simulink model "P4_Wk3"  (R2024b)
settings: Solver=ode4  StartTime=0.0  StopTime=3000  FixedStep=1  RelTol=1e-3
undefined symbols (not defined in the file or in its folder): CD, datBat, datMotor, TD, track
libraries: slpidlib x1
settings Model: Creator=brekw  LastModifiedBy=brekw
settings DebuggingCC: AlgebraicLoopMsg=none

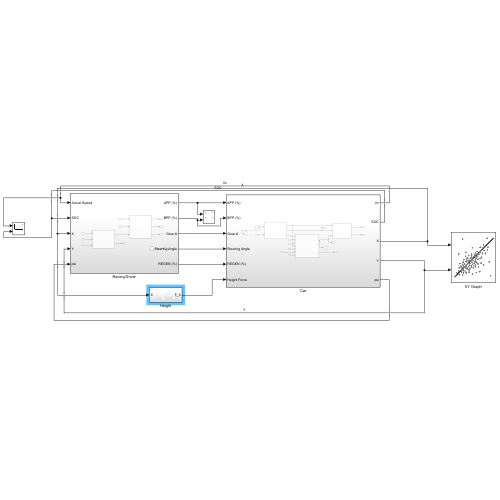
[thumbnail: Simulink's stored preview of the top-level diagram]
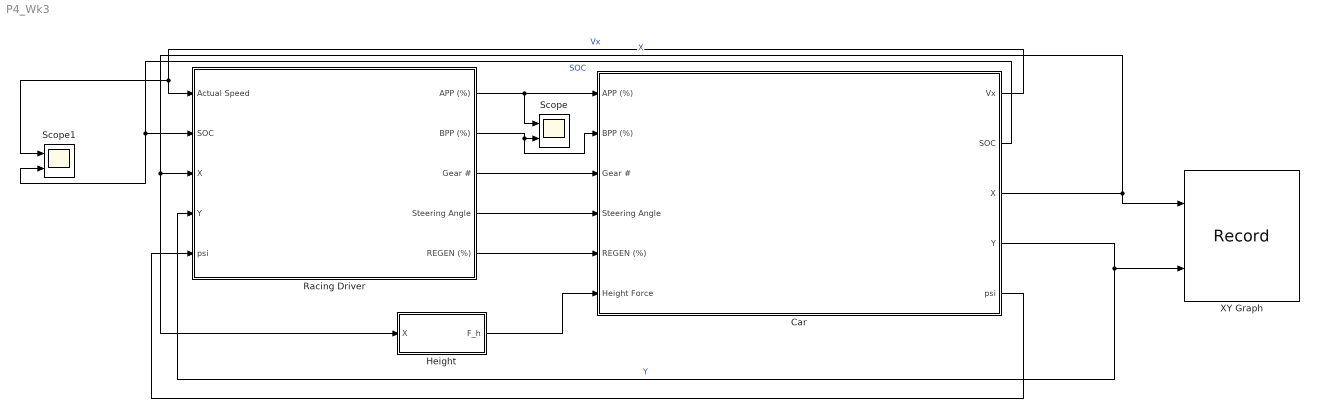
== system P4_Wk3 ==
  Car : Subsystem
  Height : Subsystem
  Racing Driver : Subsystem
  Scope : Scope  NumInputPorts=2
  Scope1 : Scope  NumInputPorts=2
  XY Graph : Record  FileSettingsInternal="{\"entries\":[{\"content\":{\"excelSettings\":{\"content\":{},\"type\":\"Streamout.ExcelSettings\"}},\"type\":\"Streamout.FileSettingStorage\",\"uuid\":\"\"}],\"packageUris\":[\"http:\\/\\/schema.mathworks.com\\/mf0\\/streamout_blocks\\/R2020a\"],\"version\":\"1.0\"}"  Layout=[1 1]  SignalsInternal="{\"entries\":[{\"content\":{\"signals\":[{\"content\":{\"blockPath\":[],\"dimensions\":[1],\"domain\":\"\",\"lineColor\":\"#a2142f\",\"plots\":[ 1 ],\"port\":1,\"sid\":[\"\"],\"signalID\":1,\"signalName\":\"X\"},\"type\":\"RecordBlkView.Signal\",\"uuid\":\"\"},{\"content\":{\"blockPath\":[],\"dimensions\":[1],\"domain\":\"\",\"lineColor\":\"#139fff\",\"plots\":[ 1 ],\"port\":2,\"sid\":[\"\"],\"signalID\":2,\"signalName\":\"Y\"},\"type\":\"RecordBlkView.Signal\",\"uuid\":\"\"}]},\"type\":\"RecordBlkView.InputSignals\",\"uuid\":\"\"}],\"packageUris\":[\"http:\\/\\/schema.mathworks.com\\/mf0\\/streamout_blocks\\/R2020a\"],\"version\":\"1.0\"}"  VisualizationBindings="{\"xyplotplugin\":{\"info\":[{\"series\":[{\"bindingParametersList\":[{\"parameter\":\"X-Axis\",\"signalID\":1,\"signalName\":\"X\"},{\"parameter\":\"Y-Axis\",\"signalID\":2,\"signalName\":\"Y\"}],\"seriesID\":0}],\"subplotID\":1}]}}"  CompatibilityTag=XY
  wires:
  Car/3(X) -> XY Graph/1, Height/1(X), Racing Driver/3(X)  "X"
  Car/4(Y) -> XY Graph/2, Racing Driver/4(Y)  "Y"
  Racing Driver/4(Steering Angle) -> Car/4(Steering Angle)
  Racing Driver/3(Gear #) -> Car/3(Gear #)
  Racing Driver/2(BPP (%)) -> Car/2(BPP (%)), Scope/2
  Racing Driver/1(APP (%)) -> Scope/1, Car/1(APP (%))
  Car/1(Vx) -> Scope1/1, Racing Driver/1(Actual Speed)  "Vx"
  Car/2(SOC) -> Scope1/2, Racing Driver/2(SOC)  "SOC"
  Racing Driver/5(REGEN (%)) -> Car/5(REGEN (%))
  Car/5(psi) -> Racing Driver/5(psi)
  Height/1(F_h) -> Car/6(Height Force)

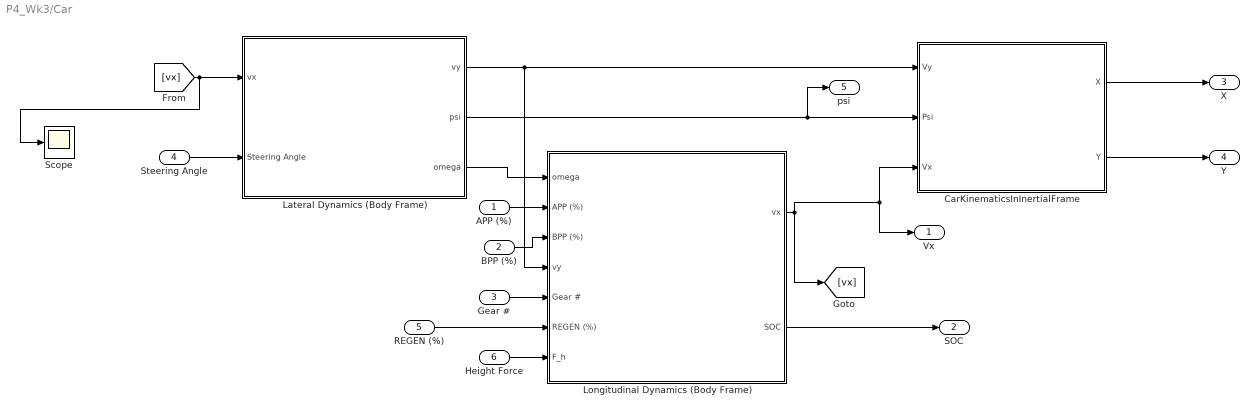
== system P4_Wk3/Car ==
  APP (%) : Inport
  BPP (%) : Inport  Port=2
  Gear # : Inport  Port=3
  Steering Angle : Inport  Port=4
  REGEN (%) : Inport  Port=5
  Height Force : Inport  Port=6
  CarKinematicsInInertialFrame : Subsystem
  Lateral Dynamics (Body Frame) : Subsystem
  Longitudinal Dynamics (Body Frame) : Subsystem
  Scope : Scope
  Vx : Outport
  SOC : Outport  Port=2
  X : Outport  Port=3
  Y : Outport  Port=4
  psi : Outport  Port=5
  wires:
  CarKinematicsInInertialFrame/1(X) -> X/1
  CarKinematicsInInertialFrame/2(Y) -> Y/1
  Lateral Dynamics (Body Frame)/1(vy) -> CarKinematicsInInertialFrame/1(Vy), Longitudinal Dynamics (Body Frame)/4(vy)
  Lateral Dynamics (Body Frame)/2(psi) -> psi/1, CarKinematicsInInertialFrame/2(Psi)
  Steering Angle/1 -> Lateral Dynamics (Body Frame)/2(Steering Angle)
  Longitudinal Dynamics (Body Frame)/1(vx) -> CarKinematicsInInertialFrame/3(Vx), Vx/1, [vx]
  Longitudinal Dynamics (Body Frame)/2(SOC) -> SOC/1
  Lateral Dynamics (Body Frame)/3(omega) -> Longitudinal Dynamics (Body Frame)/1(omega)
  [vx] -> Scope/1, Lateral Dynamics (Body Frame)/1(vx)
  Gear #/1 -> Longitudinal Dynamics (Body Frame)/5(Gear #)
  BPP (%)/1 -> Longitudinal Dynamics (Body Frame)/3(BPP (%))
  APP (%)/1 -> Longitudinal Dynamics (Body Frame)/2(APP (%))
  REGEN (%)/1 -> Longitudinal Dynamics (Body Frame)/6(REGEN (%))
  Height Force/1 -> Longitudinal Dynamics (Body Frame)/7(F_h)

== system P4_Wk3/Height ==
  X : Inport
  Constant : Constant  Value=CD.Mass
  Elevation Profile : MATLAB Function  TreatAsAtomicUnit=on
  Height Force : MATLAB Function  TreatAsAtomicUnit=on
  Scope : Scope
  F_h : Outport
  wires:
  Height Force/1(F) -> F_h/1
  X/1 -> Elevation Profile/1(x)
  Elevation Profile/2(theta) -> Height Force/2(theta)
  Constant/1 -> Height Force/1(m)
  Elevation Profile/1(h) -> Scope/1

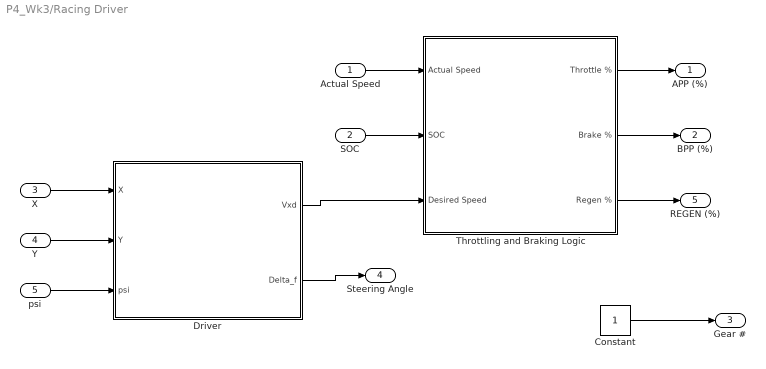
== system P4_Wk3/Racing Driver ==
  Actual Speed : Inport
  SOC : Inport  Port=2
  X : Inport  Port=3
  Y : Inport  Port=4
  psi : Inport  Port=5
  Constant : Constant
  Driver : Subsystem
  Throttling and Braking Logic : Subsystem
  APP (%) : Outport
  BPP (%) : Outport  Port=2
  Gear # : Outport  Port=3
  Steering Angle : Outport  Port=4
  REGEN (%) : Outport  Port=5
  wires:
  Constant/1 -> Gear #/1
  Driver/2(Delta_f) -> Steering Angle/1
  Driver/1(Vxd) -> Throttling and Braking Logic/3(Desired Speed)
  Actual Speed/1 -> Throttling and Braking Logic/1(Actual Speed)
  SOC/1 -> Throttling and Braking Logic/2(SOC)
  Throttling and Braking Logic/1(Throttle %) -> APP (%)/1
  Throttling and Braking Logic/2(Brake %) -> BPP (%)/1
  X/1 -> Driver/1(X)
  Y/1 -> Driver/2(Y)
  Throttling and Braking Logic/3(Regen %) -> REGEN (%)/1
  psi/1 -> Driver/3(psi)

== system P4_Wk3/Car/CarKinematicsInInertialFrame ==
  Vy : Inport
  Psi : Inport  Port=2
  Vx : Inport  Port=3
  Integrator : Integrator  InitialCondition=CD.X0
  Integrator1 : Integrator  InitialCondition=CD.Y0
  Transformation Matrix : MATLAB Function  TreatAsAtomicUnit=on
  Xdot Out : ToWorkspace  VariableName=X  SaveFormat=Timeseries  SampleTime=-1
  Ydot Out : ToWorkspace  VariableName=Y  SaveFormat=Timeseries  SampleTime=-1
  X : Outport
  Y : Outport  Port=2
  wires:
  Transformation Matrix/2(Ydot) -> Integrator1/1
  Vy/1 -> Transformation Matrix/2(vy)
  Integrator/1 -> Xdot Out/1, X/1
  Psi/1 -> Transformation Matrix/3(psi)
  Integrator1/1 -> Ydot Out/1, Y/1
  Transformation Matrix/1(Xdot) -> Integrator/1
  Vx/1 -> Transformation Matrix/1(vx)

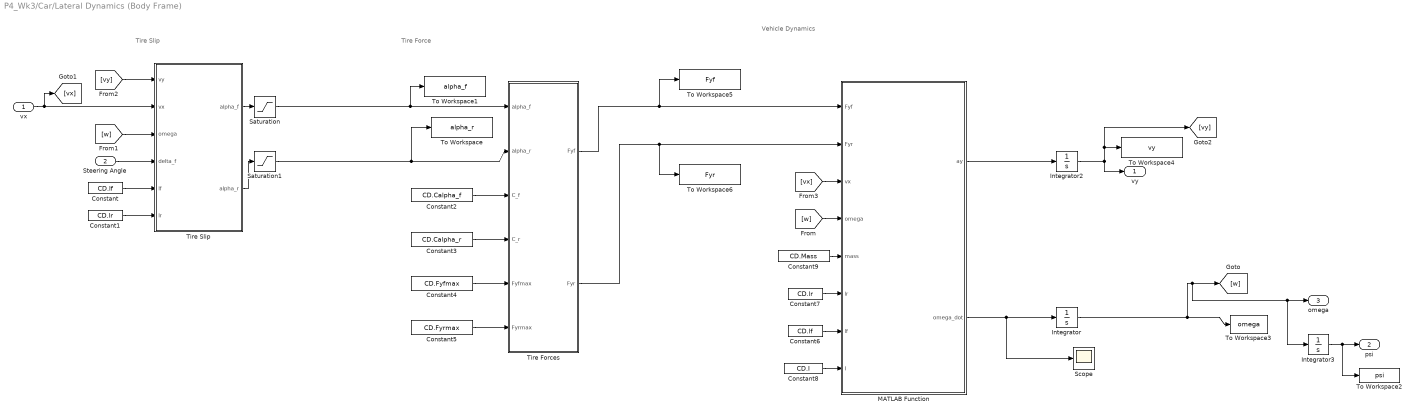
== system P4_Wk3/Car/Lateral Dynamics (Body Frame) ==
  note: Tire Slip
  note: Vehicle Dynamics
  note: Tire Force
  vx : Inport
  Steering Angle : Inport  Port=2
  Constant : Constant  Value=CD.lf
  Constant1 : Constant  Value=CD.lr
  Constant2 : Constant  Value=CD.Calpha_f
  Constant3 : Constant  Value=CD.Calpha_r
  Constant4 : Constant  Value=CD.Fyfmax
  Constant5 : Constant  Value=CD.Fyrmax
  Constant6 : Constant  Value=CD.lf
  Constant7 : Constant  Value=CD.lr
  Constant8 : Constant  Value=CD.I
  Constant9 : Constant  Value=CD.Mass
  Integrator : Integrator  InitialCondition=CD.omega0
  Integrator2 : Integrator  InitialCondition=CD.vy0
  Integrator3 : Integrator  InitialCondition=CD.psi0
  MATLAB Function : MATLAB Function  TreatAsAtomicUnit=on
  Saturation : Saturate  UpperLimit=0.01579  LowerLimit=-0.01579
  Saturation1 : Saturate  UpperLimit=0.01579  LowerLimit=-0.01579
  Scope : Scope
  Tire Forces : MATLAB Function  TreatAsAtomicUnit=on
  Tire Slip : MATLAB Function  TreatAsAtomicUnit=on
  To Workspace : ToWorkspace  VariableName=alpha_r  SaveFormat=Timeseries  SampleTime=-1
  To Workspace1 : ToWorkspace  VariableName=alpha_f  SaveFormat=Timeseries  SampleTime=-1
  To Workspace2 : ToWorkspace  VariableName=psi  SaveFormat=Timeseries  SampleTime=-1
  To Workspace3 : ToWorkspace  VariableName=omega  SaveFormat=Timeseries  SampleTime=-1
  To Workspace4 : ToWorkspace  VariableName=vy  SaveFormat=Timeseries  SampleTime=-1
  To Workspace5 : ToWorkspace  VariableName=Fyf  SaveFormat=Timeseries  SampleTime=-1
  To Workspace6 : ToWorkspace  VariableName=Fyr  SaveFormat=Timeseries  SampleTime=-1
  vy : Outport
  psi : Outport  Port=2
  omega : Outport  Port=3
  wires:
  MATLAB Function/2(omega_dot) -> Scope/1, Integrator/1
  Integrator/1 -> omega/1, Integrator3/1, [w], To Workspace3/1
  Integrator2/1 -> To Workspace4/1, [vy], vy/1
  Integrator3/1 -> psi/1, To Workspace2/1
  [w] -> MATLAB Function/4(omega)
  MATLAB Function/1(ay) -> Integrator2/1
  [vy] -> Tire Slip/1(vy)
  Saturation/1 -> To Workspace1/1, Tire Forces/1(alpha_f)
  Saturation1/1 -> To Workspace/1, Tire Forces/2(alpha_r)
  [w] -> Tire Slip/3(omega)
  Steering Angle/1 -> Tire Slip/4(delta_f)
  Tire Slip/1(alpha_f) -> Saturation/1
  Tire Slip/2(alpha_r) -> Saturation1/1
  vx/1 -> [vx], Tire Slip/2(vx)
  [vx] -> MATLAB Function/3(vx)
  Tire Forces/1(Fyf) -> To Workspace5/1, MATLAB Function/1(Fyf)
  Tire Forces/2(Fyr) -> To Workspace6/1, MATLAB Function/2(Fyr)
  Constant/1 -> Tire Slip/5(lf)
  Constant1/1 -> Tire Slip/6(lr)
  Constant2/1 -> Tire Forces/3(C_f)
  Constant3/1 -> Tire Forces/4(C_r)
  Constant4/1 -> Tire Forces/5(Fyfmax)
  Constant5/1 -> Tire Forces/6(Fyrmax)
  Constant7/1 -> MATLAB Function/6(lr)
  Constant6/1 -> MATLAB Function/7(lf)
  Constant8/1 -> MATLAB Function/8(I)
  Constant9/1 -> MATLAB Function/5(mass)

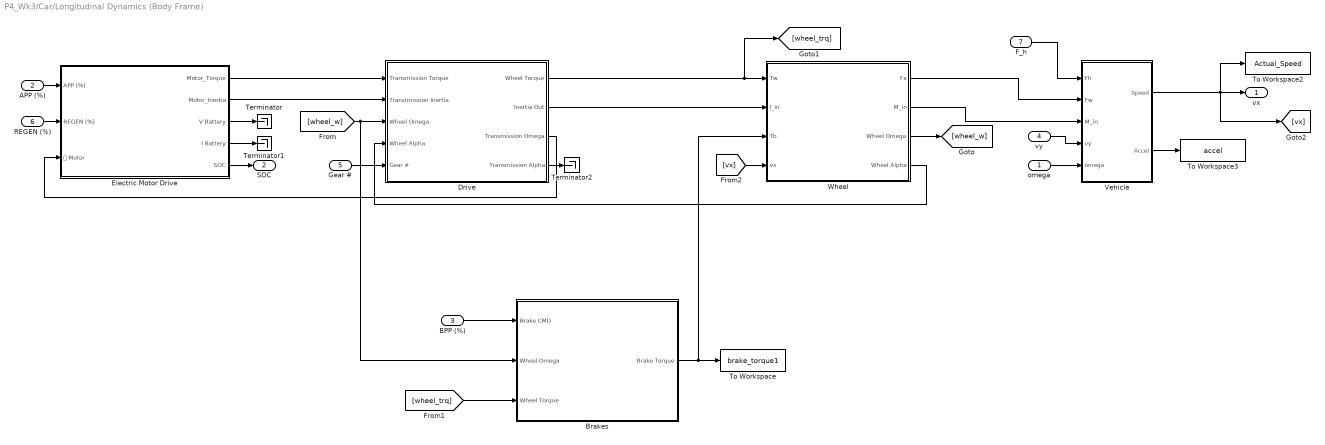
== system P4_Wk3/Car/Longitudinal Dynamics (Body Frame) ==
  omega : Inport
  APP (%) : Inport  Port=2
  BPP (%) : Inport  Port=3
  vy : Inport  Port=4
  Gear # : Inport  Port=5
  REGEN (%) : Inport  Port=6
  F_h : Inport  Port=7
  Brakes : Subsystem
  Drive : Subsystem
  Electric Motor Drive : Subsystem
  Terminator : Terminator
  Terminator1 : Terminator
  Terminator2 : Terminator
  To Workspace : ToWorkspace  VariableName=brake_torque1  SaveFormat=Timeseries  SampleTime=-1
  To Workspace2 : ToWorkspace  VariableName=Actual_Speed  SaveFormat=Timeseries  SampleTime=-1
  To Workspace3 : ToWorkspace  VariableName=accel  SaveFormat=Timeseries  SampleTime=-1
  Vehicle : Subsystem
  Wheel : Subsystem
  vx : Outport
  SOC : Outport  Port=2
  wires:
  Drive/4(Transmission Alpha) -> Terminator2/1
  Drive/2(Inertia Out) -> Wheel/2(I_in)
  [wheel_trq] -> Brakes/3(Wheel Torque)
  Electric Motor Drive/3(V Battery) -> Terminator/1
  Electric Motor Drive/2(Motor_Inertia) -> Drive/2(Transimission Inertia)
  Electric Motor Drive/1(Motor_Torque) -> Drive/1(Transmission Torque)
  Electric Motor Drive/5(SOC) -> SOC/1
  Electric Motor Drive/4(I Battery) -> Terminator1/1
  Wheel/3(Wheel Omega) -> [wheel_w]
  Drive/1(Wheel Torque) -> [wheel_trq], Wheel/1(Tw)
  [wheel_w] -> Brakes/2(Wheel Omega), Drive/3(Wheel Omega)
  BPP (%)/1 -> Brakes/1(Brake CMD)
  Drive/3(Transmission Omega) -> Electric Motor Drive/3(𝜔 Motor)
  Brakes/1(Brake Torque) -> To Workspace/1, Wheel/3(Tb)
  Wheel/2(M_in) -> Vehicle/3(M_in)
  omega/1 -> Vehicle/5(omega)
  vy/1 -> Vehicle/4(vy)
  Gear #/1 -> Drive/5(Gear #)
  APP (%)/1 -> Electric Motor Drive/1(APP (%))
  Vehicle/1(Speed) -> [vx], vx/1, To Workspace2/1
  Wheel/4(Wheel Alpha) -> Drive/4(Wheel Alpha)
  [vx] -> Wheel/4(vx)
  Vehicle/2(Accel) -> To Workspace3/1
  Wheel/1(Fx) -> Vehicle/2(Fw)
  REGEN (%)/1 -> Electric Motor Drive/2(REGEN (%))
  F_h/1 -> Vehicle/1(Fh)

== system P4_Wk3/Racing Driver/Driver ==
  X : Inport
  Y : Inport  Port=2
  psi : Inport  Port=3
  Constant5 : Constant  Value=CD.lookahead
  MATLAB Function1 : MATLAB Function  TreatAsAtomicUnit=on
  R Track : Constant  Value=TD.R
  To Workspace : ToWorkspace  VariableName=vx  SaveFormat=Timeseries  SampleTime=-1
  To Workspace1 : ToWorkspace  VariableName=delta_f  SaveFormat=Timeseries  SampleTime=-1
  carData.Length1 : Constant  Value=CD.length
  vxd in : Constant  Value=CD.vxd_straight
  Vxd : Outport
  Delta_f : Outport  Port=2
  wires:
  vxd in/1 -> To Workspace/1, Vxd/1
  X/1 -> MATLAB Function1/1(x)
  Y/1 -> MATLAB Function1/2(y)
  psi/1 -> MATLAB Function1/3(psi)
  MATLAB Function1/1(delta) -> To Workspace1/1, Delta_f/1
  carData.Length1/1 -> MATLAB Function1/4(L)
  Constant5/1 -> MATLAB Function1/5(l)
  R Track/1 -> MATLAB Function1/6(R)

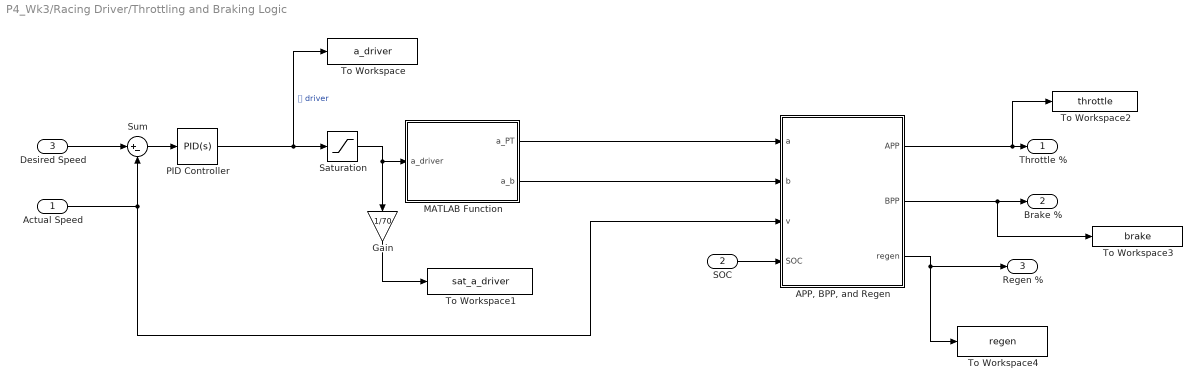
== system P4_Wk3/Racing Driver/Throttling and Braking Logic ==
  Actual Speed : Inport
  SOC : Inport  Port=2
  Desired Speed : Inport  Port=3
  "APP, BPP, and Regen" : MATLAB Function  TreatAsAtomicUnit=on
  Gain : Gain  Gain=1/70
  MATLAB Function : MATLAB Function  TreatAsAtomicUnit=on
  PID Controller : slpidlib/PID Controller  Controller=PID  Form=Parallel  TimeDomain=Continuous-time  UseExternalTs=off  SampleTime=-1  IntegratorMethod=Forward Euler  FilterMethod=Forward Euler  ControllerParametersSource=internal  P=1  I=1  UseKiTs=off  D=1  UseExternalDerivativeSource=off  N=1  UseFilter=on  TunerSelectOption=Frequency Response Based  InitialConditionSource=internal  InitialConditionForIntegrator=0  InitialConditionForFilter=0  DifferentiatorICPrevScaledInput=0  ExternalReset=none  TrackingMode=off  Kt=1  LimitOutput=off  SatLimitsSource=internal  UpperSaturationLimit=inf  LowerSaturationLimit=-inf  LinearizeAsGain=on  AntiWindupMode=none  Kb=1  LimitIntegrator=off  UpperIntegratorSaturationLimit=inf  LowerIntegratorSaturationLimit=-inf  POutMin=[]  POutMax=[]  IOutMin=[]  IOutMax=[]  DOutMin=[]  DOutMax=[]  NOutMin=[]  NOutMax=[]  SumOutMin=[]  SumOutMax=[]  SaturationOutMin=[]  SaturationOutMax=[]  PParamMin=[]  PParamMax=[]  IParamMin=[]  IParamMax=[]  DParamMin=[]  DParamMax=[]  NParamMin=[]  NParamMax=[]  KbParamMin=[]  KbParamMax=[]  KtParamMin=[]  KtParamMax=[]  KbOutMin=[]  KbOutMax=[]  KtOutMin=[]  KtOutMax=[]  IntegratorOutMin=[]  IntegratorOutMax=[]  FilterOutMin=[]  FilterOutMax=[]  SumI1OutMin=[]  SumI1OutMax=[]  SumI2OutMin=[]  SumI2OutMax=[]  SumI3OutMin=[]  SumI3OutMax=[]  SumI4OutMin=[]  SumI4OutMax=[]  SumDOutMin=[]  SumDOutMax=[]  DifferentiatorOutMin=[]  DifferentiatorOutMax=[]  FilterDiffOutCoefMin=[]  FilterDiffOutCoefMax=[]  ReciprocalOutMin=[]  ReciprocalOutMax=[]  SumDenOutMin=[]  SumDenOutMax=[]  SumNumOutMin=[]  SumNumOutMax=[]  DivideOutMin=[]  DivideOutMax=[]  UdiffTsProdOutMin=[]  UdiffTsProdOutMax=[]  NTsProdOutMin=[]  NTsProdOutMax=[]  UintegralTsProdOutMin=[]  UintegralTsProdOutMax=[]  UngainTsProdOutMin=[]  UngainTsProdOutMax=[]  ClampingZeroOutDataTypeStr=Inherit: Inherit via back propagation  ClampingZeroOutMin=[]  ClampingZeroOutMax=[]  FilterDenConstantOutDataTypeStr=Inherit: Inherit via back propagation  FilterDenConstantOutMin=[]  FilterDenConstantOutMax=[]  PCopyOutDataTypeStr=Inherit: Inherit via back propagation  PCopyOutMin=[]  PCopyOutMax=[]  NCopyOutDataTypeStr=Inherit: Inherit via back propagation  NCopyOutMin=[]  NCopyOutMax=[]  IntegratorContinuousStateAttributes=''  IntegratorStateMustResolveToSignalObject=off  IntegratorRTWStateStorageClass=Auto  FilterContinuousStateAttributes=''  FilterStateMustResolveToSignalObject=off  FilterRTWStateStorageClass=Auto  ParallelPVariant=InternalParameters  IdealPVariant=Disabled  IVariant=InternalParameters  DVariant=InternalParameters  IntegratorVariant=Continuous  SatVariant=Disabled  AWVariant=Passthrough  PCopyVariant=Disabled  TRVariant=Disabled  FdbkBlocksVariant=Forward  IdealPFdbkVariant=Disabled  SatFdbkVariant=Disabled  DerivativeFilterVariant=ContFilter  NVariant=InternalParameters  NCopyVariant=Disabled  FilterICVariant=InternalICsFilter  IntegratorICVariant=InternalICs  ExternalResetVariant=Disabled  TRSumVariant=Passthrough  SumFdbkVariant=Disabled  SumVariant=Sum_PID  TsampFilterVariant=InternalTs  TsampNgainVariant=Passthrough  TsampIntegralVariant=Disabled_SignalSpec  ExternalSaturationOutDataTypeStr=Inherit: Same as second input  DerivativeSourceVariant=ErrorSignal  PreIntVariant=InternalPreInt
  Saturation : Saturate  UpperLimit=70  LowerLimit=-70
  Sum : Sum  Inputs=|+-
  To Workspace : ToWorkspace  VariableName=a_driver  SaveFormat=Timeseries  SampleTime=-1
  To Workspace1 : ToWorkspace  VariableName=sat_a_driver  SaveFormat=Timeseries  SampleTime=-1
  To Workspace2 : ToWorkspace  VariableName=throttle  SaveFormat=Timeseries  SampleTime=-1
  To Workspace3 : ToWorkspace  VariableName=brake  SaveFormat=Timeseries  SampleTime=-1
  To Workspace4 : ToWorkspace  VariableName=regen  SaveFormat=Timeseries  SampleTime=-1
  Throttle % : Outport
  Brake % : Outport  Port=2
  Regen % : Outport  Port=3
  wires:
  PID Controller/1 -> To Workspace/1, Saturation/1  "𝛼 driver"
  Desired Speed/1 -> Sum/1
  Actual Speed/1 -> "APP, BPP, and Regen"/3(v), Sum/2
  Sum/1 -> PID Controller/1
  Saturation/1 -> Gain/1, MATLAB Function/1(a_driver)
  Gain/1 -> To Workspace1/1
  "APP, BPP, and Regen"/1(APP) -> To Workspace2/1, Throttle %/1
  "APP, BPP, and Regen"/2(BPP) -> To Workspace3/1, Brake %/1
  "APP, BPP, and Regen"/3(regen) -> Regen %/1, To Workspace4/1
  MATLAB Function/1(a_PT) -> "APP, BPP, and Regen"/1(a)
  MATLAB Function/2(a_b) -> "APP, BPP, and Regen"/2(b)
  SOC/1 -> "APP, BPP, and Regen"/4(SOC)

== system P4_Wk3/Car/Longitudinal Dynamics (Body Frame)/Brakes ==
  Brake CMD : Inport
  Wheel Omega : Inport  Port=2
  Wheel Torque : Inport  Port=3
  Constant : Constant  Value=CD.maxBrakeTorque
  Gain : Gain  Gain=CD.maxBrakeTorque/CD.radius
  MATLAB Function : MATLAB Function  TreatAsAtomicUnit=on
  Brake Torque : Outport
  wires:
  Gain/1 -> MATLAB Function/1(tau_b)
  Brake CMD/1 -> Gain/1
  MATLAB Function/1(T_b) -> Brake Torque/1
  Wheel Omega/1 -> MATLAB Function/2(w_wheel)
  Wheel Torque/1 -> MATLAB Function/3(T_wheel)
  Constant/1 -> MATLAB Function/4(maxT_b)

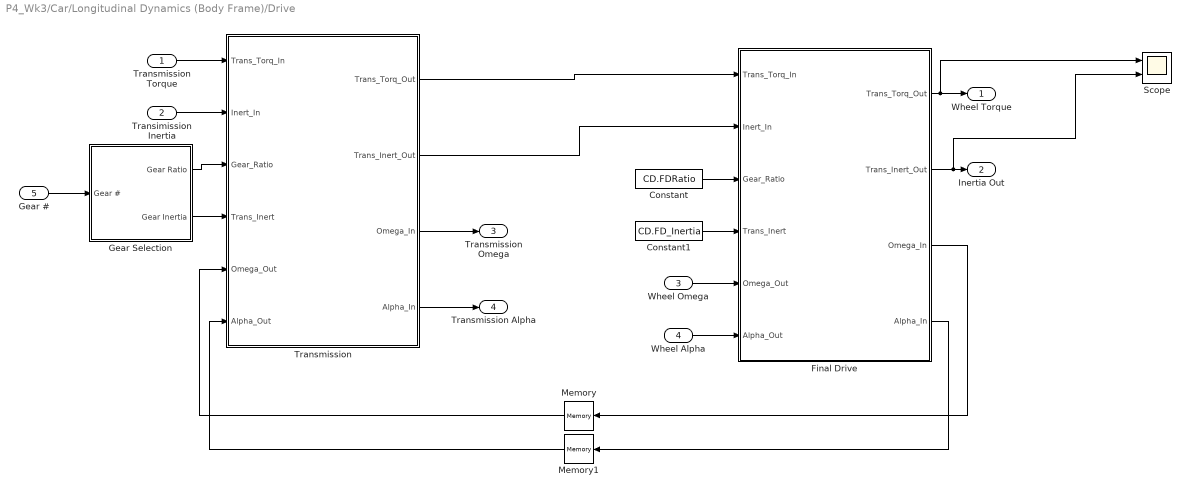
== system P4_Wk3/Car/Longitudinal Dynamics (Body Frame)/Drive ==
  Transmission Torque : Inport
  Transimission Inertia : Inport  Port=2
  Wheel Omega : Inport  Port=3
  Wheel Alpha : Inport  Port=4
  Gear # : Inport  Port=5
  Constant : Constant  Value=CD.FDRatio
  Constant1 : Constant  Value=CD.FD_Inertia
  Final Drive : MATLAB Function  TreatAsAtomicUnit=on
  Gear Selection : Subsystem
  Memory : Memory
  Memory1 : Memory
  Scope : Scope  NumInputPorts=2
  Transmission : MATLAB Function  TreatAsAtomicUnit=on
  Wheel Torque : Outport
  Inertia Out : Outport  Port=2
  Transmission Omega : Outport  Port=3
  Transmission Alpha : Outport  Port=4
  wires:
  Gear #/1 -> Gear Selection/1(Gear #)
  Gear Selection/1(Gear Ratio) -> Transmission/3(Gear_Ratio)
  Gear Selection/2(Gear Inertia) -> Transmission/4(Trans_Inert)
  Transmission Torque/1 -> Transmission/1(Trans_Torq_In)
  Transimission Inertia/1 -> Transmission/2(Inert_In)
  Wheel Omega/1 -> Final Drive/5(Omega_Out)
  Wheel Alpha/1 -> Final Drive/6(Alpha_Out)
  Transmission/1(Trans_Torq_Out) -> Final Drive/1(Trans_Torq_In)
  Transmission/2(Trans_Inert_Out) -> Final Drive/2(Inert_In)
  Transmission/4(Alpha_In) -> Transmission Alpha/1
  Transmission/3(Omega_In) -> Transmission Omega/1
  Final Drive/1(Trans_Torq_Out) -> Scope/1, Wheel Torque/1
  Final Drive/2(Trans_Inert_Out) -> Scope/2, Inertia Out/1
  Constant/1 -> Final Drive/3(Gear_Ratio)
  Constant1/1 -> Final Drive/4(Trans_Inert)
  Final Drive/4(Alpha_In) -> Memory1/1
  Final Drive/3(Omega_In) -> Memory/1
  Memory/1 -> Transmission/5(Omega_Out)
  Memory1/1 -> Transmission/6(Alpha_Out)

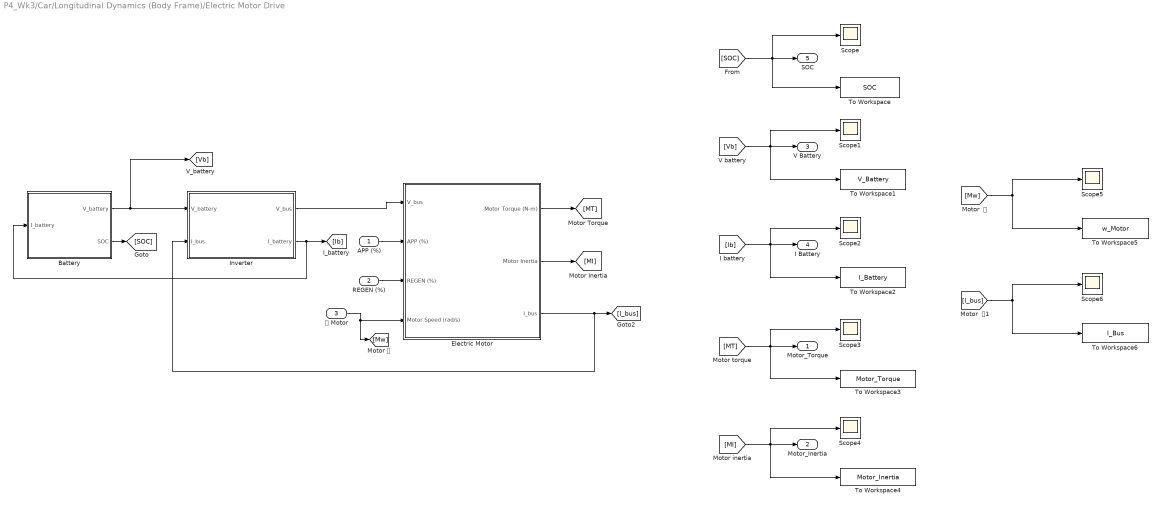
== system P4_Wk3/Car/Longitudinal Dynamics (Body Frame)/Electric Motor Drive ==
  APP (%) : Inport
  REGEN (%) : Inport  Port=2
  𝜔 Motor : Inport  Port=3
  Battery : Subsystem
  Electric Motor : Subsystem
  Inverter : Subsystem
  Scope{,1..6} (7 alike) : Scope
  To Workspace : ToWorkspace  VariableName=SOC  SaveFormat=Timeseries  SampleTime=-1
  To Workspace1 : ToWorkspace  VariableName=V_Battery  SaveFormat=Timeseries  SampleTime=-1
  To Workspace2 : ToWorkspace  VariableName=I_Battery  SaveFormat=Timeseries  SampleTime=-1
  To Workspace3 : ToWorkspace  VariableName=Motor_Torque  SaveFormat=Timeseries  SampleTime=-1
  To Workspace4 : ToWorkspace  VariableName=Motor_Inertia  SaveFormat=Timeseries  SampleTime=-1
  To Workspace5 : ToWorkspace  VariableName=w_Motor  SaveFormat=Timeseries  SampleTime=-1
  To Workspace6 : ToWorkspace  VariableName=I_Bus  SaveFormat=Timeseries  SampleTime=-1
  Motor_Torque : Outport
  Motor_Inertia : Outport  Port=2
  V Battery : Outport  Port=3
  I Battery : Outport  Port=4
  SOC : Outport  Port=5
  wires:
  Inverter/1(V_bus) -> Electric Motor/1(V_bus)
  Battery/1(V_battery) -> [Vb], Inverter/1(V_battery)
  Inverter/2(I_battery) -> Battery/1(I_battery), [Ib]
  Battery/2(SOC) -> [SOC]
  Electric Motor/3(I_bus) -> Inverter/2(I_bus), [I_bus]
  APP (%)/1 -> Electric Motor/2(APP (%))
  𝜔 Motor/1 -> Electric Motor/4(Motor Speed (rad/s)), [Mw]
  Electric Motor/1(Motor Torque (N-m)) -> [MT]
  Electric Motor/2(Motor Inertia) -> [MI]
  [SOC] -> To Workspace/1, Scope/1, SOC/1
  [Vb] -> To Workspace1/1, Scope1/1, V Battery/1
  [Ib] -> To Workspace2/1, Scope2/1, I Battery/1
  [MT] -> To Workspace3/1, Scope3/1, Motor_Torque/1
  [MI] -> To Workspace4/1, Scope4/1, Motor_Inertia/1
  [Mw] -> To Workspace5/1, Scope5/1
  [I_bus] -> To Workspace6/1, Scope6/1
  REGEN (%)/1 -> Electric Motor/3(REGEN (%))

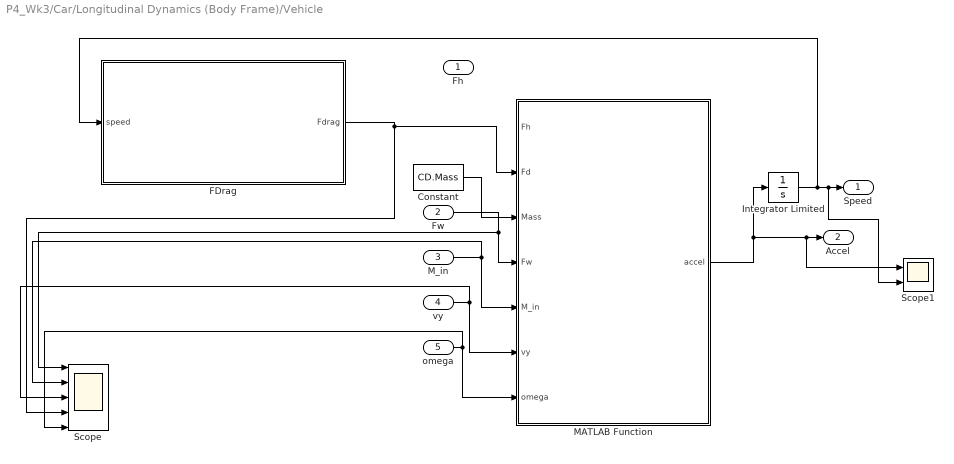
== system P4_Wk3/Car/Longitudinal Dynamics (Body Frame)/Vehicle ==
  Fh : Inport
  Fw : Inport  Port=2
  M_in : Inport  Port=3
  vy : Inport  Port=4
  omega : Inport  Port=5
  Constant : Constant  Value=CD.Mass
  FDrag : Subsystem
  Integrator Limited : Integrator  InitialCondition=CD.vx0  LimitOutput=on  UpperSaturationLimit=track.max_speed_mps  LowerSaturationLimit=0
  MATLAB Function : MATLAB Function  TreatAsAtomicUnit=on
  Scope : Scope  NumInputPorts=5
  Scope1 : Scope  NumInputPorts=2
  Speed : Outport
  Accel : Outport  Port=2
  wires:
  vy/1 -> MATLAB Function/6(vy), Scope/3
  MATLAB Function/1(accel) -> Integrator Limited/1, Scope1/1, Accel/1
  Integrator Limited/1 -> FDrag/1(speed), Scope1/2, Speed/1
  M_in/1 -> MATLAB Function/5(M_in), Scope/2
  omega/1 -> Scope/5, MATLAB Function/7(omega)
  Fw/1 -> Scope/1, MATLAB Function/4(Fw)
  FDrag/1(Fdrag) -> Scope/4, MATLAB Function/2(Fd)
  Constant/1 -> MATLAB Function/3(Mass)

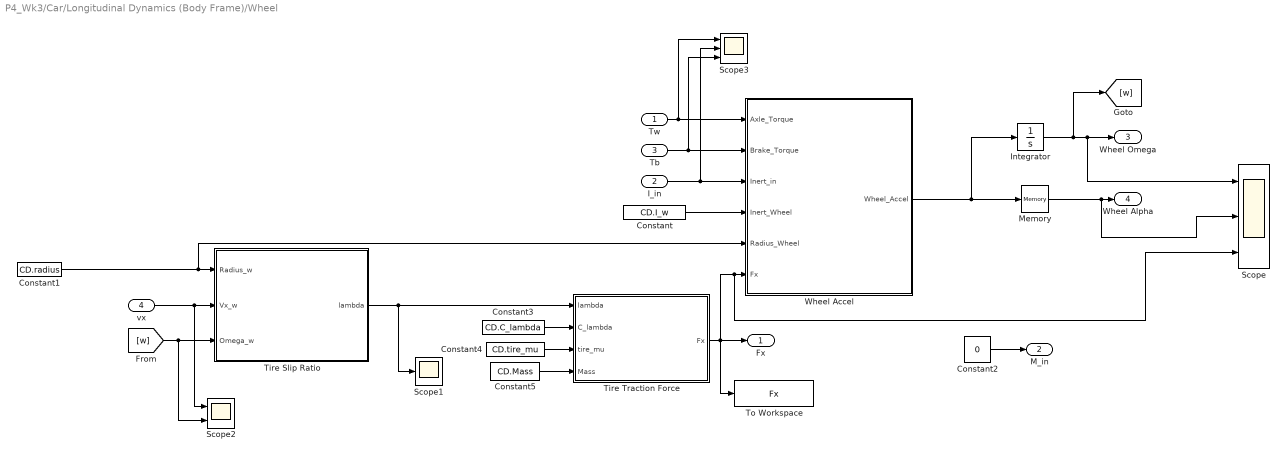
== system P4_Wk3/Car/Longitudinal Dynamics (Body Frame)/Wheel ==
  Tw : Inport
  I_in : Inport  Port=2
  Tb : Inport  Port=3
  vx : Inport  Port=4
  Constant : Constant  Value=CD.I_w
  Constant1 : Constant  Value=CD.radius
  Constant2 : Constant  Value=0
  Constant3 : Constant  Value=CD.C_lambda
  Constant4 : Constant  Value=CD.tire_mu
  Constant5 : Constant  Value=CD.Mass
  Integrator : Integrator  InitialCondition=CD.omega0
  Memory : Memory
  Scope : Scope  NumInputPorts=3
  Scope1 : Scope
  Scope2 : Scope  NumInputPorts=2
  Scope3 : Scope  NumInputPorts=3
  Tire Slip Ratio : MATLAB Function  TreatAsAtomicUnit=on
  Tire Traction Force : MATLAB Function  TreatAsAtomicUnit=on
  To Workspace : ToWorkspace  VariableName=Fx  SaveFormat=Timeseries  SampleTime=-1
  Wheel Accel : MATLAB Function  TreatAsAtomicUnit=on
  Fx : Outport
  M_in : Outport  Port=2
  Wheel Omega : Outport  Port=3
  Wheel Alpha : Outport  Port=4
  wires:
  Tw/1 -> Scope3/1, Wheel Accel/1(Axle_Torque)
  Tb/1 -> Wheel Accel/2(Brake_Torque), Scope3/3
  I_in/1 -> Scope3/2, Wheel Accel/3(Inert_in)
  Constant/1 -> Wheel Accel/4(Inert_Wheel)
  Memory/1 -> Scope/2, Wheel Alpha/1
  Wheel Accel/1(Wheel_Accel) -> Integrator/1, Memory/1
  vx/1 -> Scope2/1, Tire Slip Ratio/2(Vx_w)
  Constant2/1 -> M_in/1
  [w] -> Tire Slip Ratio/3(Omega_w), Scope2/2
  Tire Slip Ratio/1(lambda) -> Scope1/1, Tire Traction Force/1(lambda)
  Constant3/1 -> Tire Traction Force/2(C_lambda)
  Tire Traction Force/1(Fx) -> To Workspace/1, Scope/3, Wheel Accel/6(Fx), Fx/1
  Constant1/1 -> Tire Slip Ratio/1(Radius_w), Wheel Accel/5(Radius_Wheel)
  Constant4/1 -> Tire Traction Force/3(tire_mu)
  Constant5/1 -> Tire Traction Force/4(Mass)
  Integrator/1 -> [w], Scope/1, Wheel Omega/1

== system P4_Wk3/Car/Longitudinal Dynamics (Body Frame)/Drive/Gear Selection ==
  Gear # : Inport
  1-D Lookup Table : Lookup_n-D  NumberOfTableDimensions=1  BreakpointsForDimension1=CD.gearNumb  Table=CD.gearRatios  InternalRulePriority=Speed  RndMeth=Simplest
  1-D Lookup Table1 : Lookup_n-D  NumberOfTableDimensions=1  BreakpointsForDimension1=CD.gearNumb  Table=CD.gearInertias  InternalRulePriority=Speed  RndMeth=Simplest
  Rate Limiter : RateLimiter  SampleTimeMode=inherited
  Rate Limiter1 : RateLimiter  SampleTimeMode=inherited
  Gear Ratio : Outport
  Gear Inertia : Outport  Port=2
  wires:
  1-D Lookup Table/1 -> Rate Limiter/1
  Rate Limiter/1 -> Gear Ratio/1
  1-D Lookup Table1/1 -> Rate Limiter1/1
  Rate Limiter1/1 -> Gear Inertia/1
  Gear #/1 -> 1-D Lookup Table1/1, 1-D Lookup Table/1

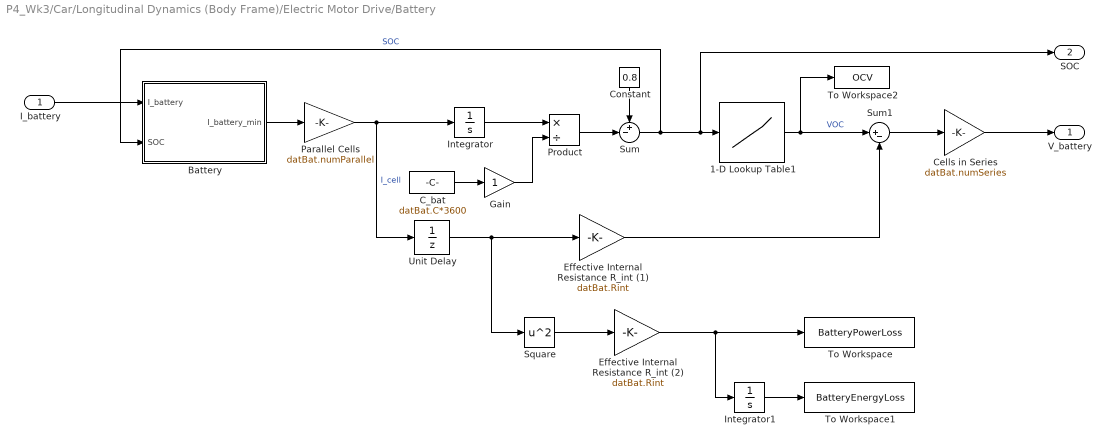
== system P4_Wk3/Car/Longitudinal Dynamics (Body Frame)/Electric Motor Drive/Battery ==
  I_battery : Inport
  1-D Lookup Table1 : Lookup_n-D  NumberOfTableDimensions=1  BreakpointsForDimension1=datBat.SOC  Table=datBat.OCV  InternalRulePriority=Speed  RndMeth=Simplest
  Battery : MATLAB Function  TreatAsAtomicUnit=on
  C_bat : Constant  Value=datBat.C*3600
  Cells in Series : Gain  Gain=datBat.numSeries
  Constant : Constant  Value=0.8
  Effective Internal Resistance R_int (1) : Gain  Gain=datBat.Rint
  Effective Internal Resistance R_int (2) : Gain  Gain=datBat.Rint
  Gain : Gain
  Integrator : Integrator
  Integrator1 : Integrator
  Parallel Cells : Gain  Gain=datBat.numParallel
  Product : Product  Inputs=*/
  Square : Math  Operator=square
  Sum : Sum  Inputs=+-|
  Sum1 : Sum  Inputs=|+-
  To Workspace : ToWorkspace  VariableName=BatteryPowerLoss  SaveFormat=Timeseries  SampleTime=-1
  To Workspace1 : ToWorkspace  VariableName=BatteryEnergyLoss  SaveFormat=Timeseries  SampleTime=-1
  To Workspace2 : ToWorkspace  VariableName=OCV  SaveFormat=Timeseries  SampleTime=-1
  Unit Delay : UnitDelay  SampleTime=-1  HasFrameUpgradeWarning=on
  V_battery : Outport
  SOC : Outport  Port=2
  wires:
  I_battery/1 -> Battery/1(I_battery)
  Battery/1(I_battery_min) -> Parallel Cells/1
  Integrator/1 -> Product/1
  Parallel Cells/1 -> Unit Delay/1, Integrator/1  "I_cell"
  C_bat/1 -> Gain/1
  Gain/1 -> Product/2
  Constant/1 -> Sum/1
  Product/1 -> Sum/2
  Sum/1 -> Battery/2(SOC), SOC/1, 1-D Lookup Table1/1  "SOC"
  1-D Lookup Table1/1 -> To Workspace2/1, Sum1/1  "VOC"
  Sum1/1 -> Cells in Series/1
  Unit Delay/1 -> Square/1, Effective Internal Resistance R_int (1)/1
  Effective Internal Resistance R_int (1)/1 -> Sum1/2
  Square/1 -> Effective Internal Resistance R_int (2)/1
  Effective Internal Resistance R_int (2)/1 -> Integrator1/1, To Workspace/1
  Integrator1/1 -> To Workspace1/1
  Cells in Series/1 -> V_battery/1

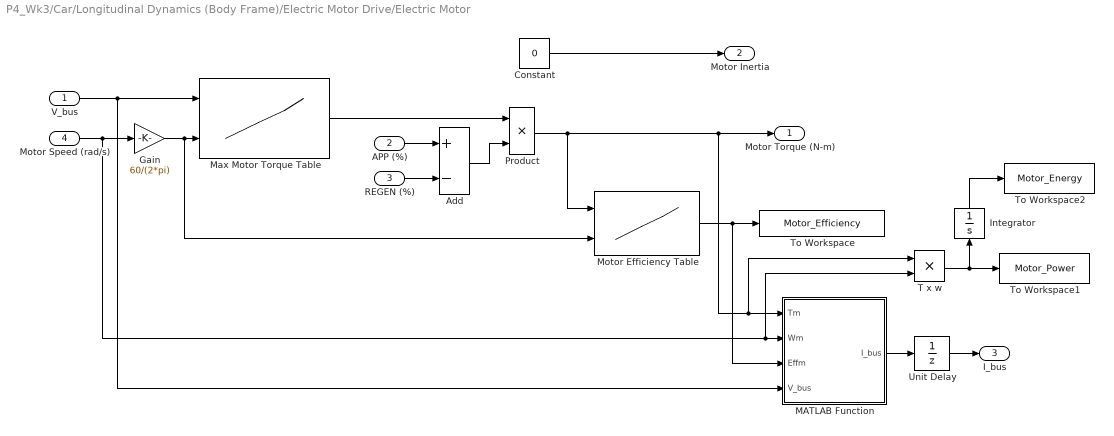
== system P4_Wk3/Car/Longitudinal Dynamics (Body Frame)/Electric Motor Drive/Electric Motor ==
  V_bus : Inport
  APP (%) : Inport  Port=2
  REGEN (%) : Inport  Port=3
  Motor Speed (rad/s) : Inport  Port=4
  Add : Sum  Inputs=+-
  Constant : Constant  Value=0
  Gain : Gain  Gain=60/(2*pi)
  Integrator : Integrator
  MATLAB Function : MATLAB Function  TreatAsAtomicUnit=on
  Max Motor Torque Table : Lookup_n-D  BreakpointsForDimension1=datMotor.vbus  BreakpointsForDimension2=datMotor.rpm  Table=datMotor.maxtorque  InternalRulePriority=Speed  RndMeth=Simplest
      settings: InputPortMap=u0,u1
  Motor Efficiency Table : Lookup_n-D  BreakpointsForDimension1=datMotor.eta_torque  BreakpointsForDimension2=datMotor.eta_speed  Table=datMotor.eta_val  InternalRulePriority=Speed  RndMeth=Simplest
      settings: InputPortMap=u0,u1
  Product : Product
  T x w : Product
  To Workspace : ToWorkspace  VariableName=Motor_Efficiency  SaveFormat=Timeseries  SampleTime=-1
  To Workspace1 : ToWorkspace  VariableName=Motor_Power  SaveFormat=Timeseries  SampleTime=-1
  To Workspace2 : ToWorkspace  VariableName=Motor_Energy  SaveFormat=Timeseries  SampleTime=-1
  Unit Delay : UnitDelay  SampleTime=-1  HasFrameUpgradeWarning=on
  Motor Torque (N-m) : Outport
  Motor Inertia : Outport  Port=2
  I_bus : Outport  Port=3
  wires:
  V_bus/1 -> MATLAB Function/4(V_bus), Max Motor Torque Table/1
  Motor Speed (rad/s)/1 -> Gain/1, T x w/2, MATLAB Function/2(Wm)
  Max Motor Torque Table/1 -> Product/1
  Product/1 -> Motor Efficiency Table/1, Motor Torque (N-m)/1, MATLAB Function/1(Tm), T x w/1
  Constant/1 -> Motor Inertia/1
  Motor Efficiency Table/1 -> MATLAB Function/3(Effm), To Workspace/1
  MATLAB Function/1(I_bus) -> Unit Delay/1
  Unit Delay/1 -> I_bus/1
  T x w/1 -> Integrator/1, To Workspace1/1
  Integrator/1 -> To Workspace2/1
  Gain/1 -> Motor Efficiency Table/2, Max Motor Torque Table/2
  APP (%)/1 -> Add/1
  REGEN (%)/1 -> Add/2
  Add/1 -> Product/2

== system P4_Wk3/Car/Longitudinal Dynamics (Body Frame)/Electric Motor Drive/Inverter ==
  V_battery : Inport
  I_bus : Inport  Port=2
  Inverter Efficiency : Constant  Value=0.95
  MATLAB Function : MATLAB Function  TreatAsAtomicUnit=on
  V_bus : Outport
  I_battery : Outport  Port=2
  wires:
  V_battery/1 -> MATLAB Function/1(V_battery)
  Inverter Efficiency/1 -> MATLAB Function/2(Eff_Inv)
  I_bus/1 -> MATLAB Function/3(I_bus)
  MATLAB Function/1(V_bus) -> V_bus/1
  MATLAB Function/2(I_battery) -> I_battery/1

== system P4_Wk3/Car/Longitudinal Dynamics (Body Frame)/Vehicle/FDrag ==
  speed : Inport
  Drag Force : MATLAB Function  TreatAsAtomicUnit=on
  To Workspace : ToWorkspace  VariableName=Fdrag  SaveFormat=Timeseries  SampleTime=-1
  drag coeff : Constant  Value=CD.C2
  rolling friciton : Constant  Value=CD.C1
  static friction : Constant  Value=CD.C0
  Fdrag : Outport
  wires:
  drag coeff/1 -> Drag Force/3(C2)
  static friction/1 -> Drag Force/1(C0)
  Drag Force/1(Fdrag) -> Fdrag/1, To Workspace/1
  rolling friciton/1 -> Drag Force/2(C1)
  speed/1 -> Drag Force/4(v)

== matlab function P4_Wk3/Car/Longitudinal Dynamics (Body Frame)/Vehicle/FDrag/Drag Force ==
  data: C0 input; Fdrag output; C1 input; C2 input; v input
function Fdrag = fcn(C0, C1, C2, v)

Fdrag = C0 + C1 * abs(v) + C2 * abs(v)^2;

== matlab function P4_Wk3/Car/Longitudinal Dynamics (Body Frame)/Wheel/Wheel Accel ==
  data: Axle_Torque input; Wheel_Accel output; Brake_Torque input; Inert_in input; Inert_Wheel input; Radius_Wheel input; Fx input
function Wheel_Accel = fcn(Axle_Torque, Brake_Torque, Inert_in, Inert_Wheel, Radius_Wheel, Fx)

% Wheel Acceleration (rad/s^2)
Wheel_Accel = (Axle_Torque - Brake_Torque - (Fx * Radius_Wheel)) / (Inert_in + Inert_Wheel);

== matlab function P4_Wk3/Car/CarKinematicsInInertialFrame/Transformation Matrix ==
  data: vx input; Xdot output; vy input; psi input; Ydot output
function [Xdot, Ydot] = fcn(vx, vy, psi)
    R_M_neg = [cos(psi) -sin(psi);
               sin(psi) cos(psi)];

    Matrix_Result = R_M_neg * [vx; vy];
    Xdot = Matrix_Result(1);
    Ydot = Matrix_Result(2);
end

== matlab function P4_Wk3/Car/Longitudinal Dynamics (Body Frame)/Wheel/Tire Slip Ratio ==
  data: Radius_w input; lambda output; Vx_w input; Omega_w input
function lambda = fcn(Radius_w, Vx_w, Omega_w)

% Arbitrary Constant
e = 0.01;

% Tire Slip Ratio
lambda = (Radius_w * Omega_w - Vx_w) / (Radius_w * Omega_w + e ^ (-abs(Omega_w)));

== matlab function P4_Wk3/Car/Longitudinal Dynamics (Body Frame)/Wheel/Tire Traction Force ==
  data: lambda input; C_lambda input; Fx output; tire_mu input; Mass input
function Fx = fcn(lambda, C_lambda, tire_mu, Mass)

% Longitudinal Force (N)
Fx = (C_lambda * tire_mu * Mass * 9.81 * lambda) * lambda;

== matlab function P4_Wk3/Racing Driver/Throttling and Braking Logic/MATLAB Function ==
  data: a_driver input; a_PT output; a_b output
function [a_PT, a_b]= fcn(a_driver)

% 𝛼_driver < 0
if a_driver < 0
    a_PT = 0;
    a_b = -a_driver;

% 𝛼_driver ≥ 0
else
    a_PT = a_driver;
    a_b = 0; 

end

== matlab function P4_Wk3/Racing Driver/Throttling and Braking Logic/APP, BPP, and Regen ==
  data: a input; APP output; b input; v input; SOC input; BPP output; regen output
function [APP, BPP, regen] = fcn(a, b, v, SOC)

% Friction Breaking is 100% when v < 5 mph
if v < (5*(1609.34/3600))
    regen = 0;
    friction = 1;
    APP = a;
    BPP = b;

% When speed >= 25 mph friction braking is only 5%
elseif v >= (25*(1609.34/3600))
    regen = 0.95;
    friction = 0.05;
    APP = a;
    BPP = b*friction;

% Friction breaking varies between 5mph and 25 mph
else
    regen = (0.95/20)*v;
    friction = 1 - regen;
    APP = a;
    BPP = b*friction;

end

% If SOC drops below 10% then the vehicle stops
if SOC <= 0.1
    APP = 0;
    BPP = b;
    regen = 0;

% If SOC goes above 95% regen stops charging
elseif SOC > 0.95
    regen = 0;

end

== matlab function P4_Wk3/Height/Elevation Profile ==
  data: h output; x input; theta output
function [h, theta]  = fcn(x)

h = exp((x-450)/50)/(1+exp((x-450)/50)) * 10;
dh = (10/50) * exp((x - 450)/50) / (1 + exp((x - 450)/50))^2;

theta = atan(dh); % Slope Angle in Radians

== matlab function P4_Wk3/Height/Height Force ==
  data: m input; F output; theta input
function F = fcn(m, theta)

F = m * 9.81 * sin(theta);

== matlab function P4_Wk3/Car/Lateral Dynamics (Body Frame)/Tire Forces ==
  data: alpha_f input; Fyf output; alpha_r input; Fyr output; C_f input; C_r input; Fyfmax input; Fyrmax input
function [Fyf, Fyr]= fcn(alpha_f, alpha_r, C_f, C_r, Fyfmax, Fyrmax)

% Front Tire Force (N)
Fyf = min(Fyfmax, C_f*alpha_f);

% Rear Tire Force (N)
Fyr = min(Fyrmax, C_r*alpha_r);

== matlab function P4_Wk3/Racing Driver/Driver/MATLAB Function1 ==
  data: x input; delta output; y input; psi input; L input; l input; R input
function delta = pure_pursuit_feedforward(x, y, psi, L, l, R)

% Determine Lookahead Point
if (y < 50) && (x >= 0) && (x <= 900) % Bottom straight
    if x + l <= 900
        x_l = x + l;
        y_l = 0;
    else
        straight_part = 900 - x;
        curve_part = l - straight_part;
        theta = curve_part / R;
        x_l = 900 + R * cos(theta);
        y_l = 200 + R * sin(theta);
    end
elseif (y > 350) && (x >= 0) && (x <= 900) % Top straight
    if x - l >= 0
        x_l = x - l;
        y_l = 400;
    else
        straight_part = x;
        curve_part = l - straight_part;
        theta = curve_part / R;
        x_l = 0 + R * cos(pi - theta);
        y_l = 200 + R * sin(pi - theta);
    end

elseif (x > 900) && (y >= 0) && (y <= 400) % Right curve
    theta_vehicle = atan2(y - 200, x - 900);
    arc_length_traveled = R * theta_vehicle;
    theta_total = (arc_length_traveled + l) / R;
    x_l = 900 + R * cos(theta_total);
    y_l = 200 + R * sin(theta_total);

elseif (x < 0) && (y >= 0) && (y <= 400) % Left curve
    theta_vehicle = atan2(y - 200, x);
    arc_length_traveled = R * (pi - theta_vehicle);
    theta_total = (arc_length_traveled + l) / R;
    x_l = 0 + R * cos(pi - theta_total);
    y_l = 200 + R * sin(pi - theta_total);

else
    x_l = x + l;
    y_l = y;
end

% Calculate desired heading
psi_d = atan2(y_l - y, x_l - x);

% Calculate heading error
alpha = psi_d - psi;

alpha = atan2(sin(alpha), cos(alpha));

delta_pure_pursuit = atan2(2 * L * sin(alpha), l);

%Apply smoothing gain to prevent oscillations
steering_gain = 0.6; 
delta = steering_gain * delta_pure_pursuit;

end

== matlab function P4_Wk3/Car/Longitudinal Dynamics (Body Frame)/Brakes/MATLAB Function ==
  data: tau_b input; T_b output; w_wheel input; T_wheel input; maxT_b input
function T_b = fcn(tau_b, w_wheel, T_wheel, maxT_b)
    
    maxTotalTorque = 6000;   % Nm (tunable safety limit)

    % Brake torque to max allowed
    T_b = max(min(tau_b, maxT_b), 0);

    % Disable braking at zero speed
    if abs(w_wheel) < 0.1
        T_b = 0;
    end

    % Torque limit logic (ABS)
    if abs(T_b + T_wheel) > maxTotalTorque
        T_b = maxTotalTorque - abs(T_wheel);
        T_b = max(T_b, 0); % prevent negative torque
    end
end

== matlab function P4_Wk3/Car/Longitudinal Dynamics (Body Frame)/Electric Motor Drive/Battery/Battery ==
  data: I_battery input; I_battery_min output; SOC input
function I_battery_min = fcn(I_battery, SOC)

    if SOC <= 0.1
	  I_battery_min = 0;
    else
	  I_battery_min = I_battery;
    end
    
end

== matlab function P4_Wk3/Car/Longitudinal Dynamics (Body Frame)/Electric Motor Drive/Electric Motor/MATLAB Function ==
  data: Tm input; I_bus output; Wm input; Effm input; V_bus input
function I_bus = fcn(Tm, Wm, Effm, V_bus)

% Driving Mode
if Tm >= 0
    P_mech = Tm * Wm;                            
    I_bus = P_mech / (Effm * V_bus);

% Regen Mode
else
    P_mech = abs(Tm * Wm);                        
    I_bus = -P_mech * Effm / V_bus;               
end

== matlab function P4_Wk3/Car/Longitudinal Dynamics (Body Frame)/Electric Motor Drive/Inverter/MATLAB Function ==
  data: V_battery input; V_bus output; Eff_Inv input; I_bus input; I_battery output
function [V_bus, I_battery] = fcn(V_battery, Eff_Inv, I_bus)

    V_bus = V_battery;
    P_bus = V_bus * I_bus;
    sgn_P_bus = P_bus / (abs(P_bus) + 0.001);

    if V_battery > 1
        I_battery = (P_bus / Eff_Inv^sgn_P_bus) / V_battery;
    else
        I_battery = 0;
    end

end

== matlab function P4_Wk3/Car/Lateral Dynamics (Body Frame)/Tire Slip ==
  data: vy input; alpha_f output; vx input; omega input; delta_f input; alpha_r output; lf input; lr input
function [alpha_f, alpha_r]= fcn(vy, vx, omega, delta_f, lf, lr)


if vx ~= 0

    % Front Tire Slip (rads)
    alpha_f = delta_f - (vy + lf*omega) / vx;

    % Rear Tire Slip (rads)
    alpha_r = - (vy - lr*omega) / vx;

else

    alpha_r = 0;
    alpha_f = 0;

end

== matlab function P4_Wk3/Car/Lateral Dynamics (Body Frame)/MATLAB Function ==
  data: Fyf input; Fyr input; vx input; omega input; ay output; omega_dot output; mass input; lr input; lf input; I input
function [ay, omega_dot]= fcn(Fyf, Fyr, vx, omega, mass, lr, lf, I)

Fynet = Fyf + Fyr;

Mnet = Fyf * lf - Fyr * lr;

% Linear Acceleration (m/s^2)
ay = Fynet / mass - omega * vx;


% Angular Acceleration (rad/^2)
omega_dot = Mnet / I;

== matlab function P4_Wk3/Car/Longitudinal Dynamics (Body Frame)/Drive/Transmission ==
  data: Trans_Torq_In input; Trans_Torq_Out output; Inert_In input; Gear_Ratio input; Trans_Inert input; Omega_Out input; Alpha_Out input; Trans_Inert_Out output; Omega_In output; Alpha_In output
function [Trans_Torq_Out, Trans_Inert_Out, Omega_In, Alpha_In] = fcn(Trans_Torq_In, Inert_In, Gear_Ratio, Trans_Inert, Omega_Out, Alpha_Out)

% Torque (Nm)
Trans_Torq_Out = Trans_Torq_In * Gear_Ratio;

% Inertia (kg*m^2
Trans_Inert_Out = (Inert_In + Trans_Inert) * Gear_Ratio ^ 2;

% Transmission Radial Velocity (rad/s)
Omega_In = Omega_Out * Gear_Ratio;

% Transmission Radial Acceleration (rad/s^2)
Alpha_In = Alpha_Out * Gear_Ratio;

== matlab function P4_Wk3/Car/Longitudinal Dynamics (Body Frame)/Vehicle/MATLAB Function ==
  data: Fh input; accel output; Fd input; Mass input; Fw input; M_in input; vy input; omega input
function accel = Vehicle(Fh, Fd, Mass, Fw, M_in, vy, omega)

% Vehicle Acceleration (m/s^2)
accel = ((Fw - Fd - Fh) / (Mass + M_in)) + vy * omega;

== matlab function P4_Wk3/Car/Longitudinal Dynamics (Body Frame)/Drive/Final Drive ==
  data: Trans_Torq_In input; Trans_Torq_Out output; Inert_In input; Gear_Ratio input; Trans_Inert input; Omega_Out input; Alpha_Out input; Trans_Inert_Out output; Omega_In output; Alpha_In output
function [Trans_Torq_Out, Trans_Inert_Out, Omega_In, Alpha_In] = fcn(Trans_Torq_In, Inert_In, Gear_Ratio, Trans_Inert, Omega_Out, Alpha_Out)

% Torque (Nm)
Trans_Torq_Out = Trans_Torq_In * Gear_Ratio;

% Inertia (kg*m^2
Trans_Inert_Out = (Inert_In + Trans_Inert) * Gear_Ratio ^ 2;

% Transmission Radial Velocity (rad/s)
Omega_In = Omega_Out * Gear_Ratio;

% Transmission Radial Acceleration (rad/s^2)
Alpha_In = Alpha_Out * Gear_Ratio;
